simulink model "model_3dof_24"  (R2024b)
settings: Solver=ode4  StartTime=0.0  StopTime=10.0  FixedStep=0.001  RelTol=1e-3
model workspace: external: MATLAB File params.m (data not in the file)
values from neighbouring files (symbols this model uses):
  A = [ ... (first row only)    [params.m]    (also in params_1dof.m; params_3dof.m)
  B = [ ... (first row only)    [params.m]    (also in params_1dof.m = [0; 1/I_xx]; params_3dof.m)
  C = [ ... (first row only)    [params.m]    (also in params_1dof.m = [1 0]; params_3dof.m)
  D = [ ... (first row only)    [params.m]    (also in params_3dof.m)
settings Model: Creator=schwmaxi  LastModifiedBy=schwmaxi
settings OptimizationCC: UseDivisionForNetSlopeComputation=on  GainParamInheritBuiltInType=on  UseFloatMulNetSlope=on  EnhancedBackFolding=on  BooleansAsBitfields=on  PassReuseOutputArgsAs=Individual arguments  StateBitsets=on  DataBitsets=on  ZeroExternalMemoryAtStartup=off  ZeroInternalMemoryAtStartup=off  NoFixptDivByZeroProtection=on  EfficientFloat2IntCast=on  LifeSpan=1  OptimizeBlockOrder=speed  DifferentSizesBufferReuse=on  EfficientTunableParamExpr=on
settings DebuggingCC: ParameterTunabilityLossMsg=error
settings HardwareCC: ProdBitPerPointer=32  ProdBitPerSizeT=32  ProdBitPerPtrDiffT=32  ProdLargestAtomicFloat=None  ProdWordSize=32  ProdLongLongMode=on  ProdHWDeviceType=Custom Processor->Custom Processor
settings SFSimCC: MATLABDynamicMemAlloc=off  SimTargetLang=C++
settings RTWCC: Description=Embedded Coder  SystemTargetFile=ert.tlc  GenCodeOnly=on  TemplateMakefile=ert_default_tmf  TargetLang=C++
settings CodeAppCC: ForceParamTrailComments=on  IgnoreCustomStorageClasses=off  OperatorAnnotations=on  SimulinkDataObjDesc=on  SFDataObjDesc=on  CustomSymbolStrGlobalVar=rt$N$M  CustomSymbolStrType=$N$M  CustomSymbolStrFcn=$N$M$F  CustomSymbolStrMacro=$N$M  InsertBlockDesc=on
settings ERTTargetCC: TargetLangStandard=C++11 (ISO)  GenerateSampleERTMain=on  IncludeMdlTerminateFcn=off  CombineSignalStateStructs=on  SupportAbsoluteTime=off  CodeInterfacePackaging=C++ class  SupportComplex=off  SupportNonInlinedSFcns=on  InlinedParameterPlacement=Hierarchical  RootIOFormat=Structure reference  ERTCustomFileTemplate=example_file_process.tlc  ERTFilePackagingFormat=CompactWithDataFile

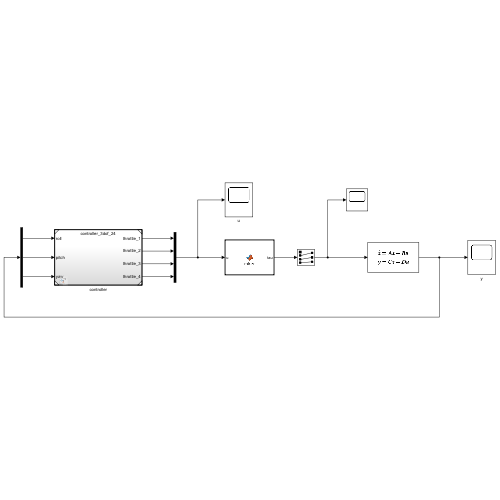
[thumbnail: Simulink's stored preview of the top-level diagram]
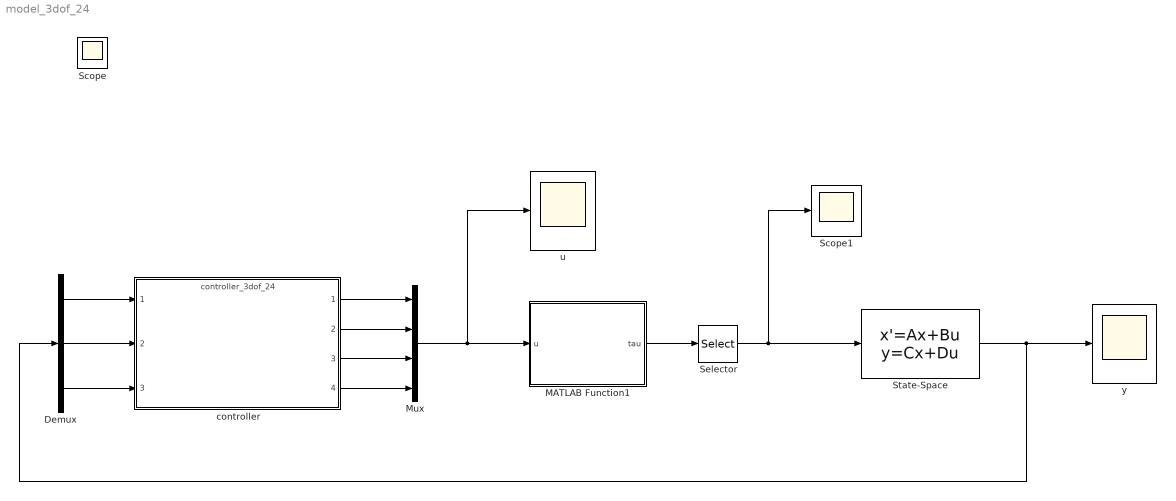
== system model_3dof_24 ==
  Demux : Demux  Outputs=3
  MATLAB Function1 : MATLAB Function  TreatAsAtomicUnit=on
  Mux : Mux
  Scope1 : Scope
  Selector : Selector  InputPortWidth=4  IndexOptions=Index vector (dialog)  Indices=[2 3 4]  OutputSizes=1
  State-Space : StateSpace  A=A  B=B  C=C  D=D  InitialCondition=[0.5, 0, 0, 0, 0, 0]'
  controller : ModelReference  ModelNameDialog=controller_3dof_24.slx  SimulationMode=Normal  ModelReferenceVersion=1.1
  u : Scope
  y : Scope
  Scope : Scope
  wires:
  MATLAB Function1/1(tau) -> Selector/1
  controller/2 -> Mux/2
  controller/1 -> Mux/1
  controller/3 -> Mux/3
  controller/4 -> Mux/4
  Mux/1 -> u/1, MATLAB Function1/1(u)
  Demux/2 -> controller/2
  Demux/1 -> controller/1
  Demux/3 -> controller/3
  Selector/1 -> State-Space/1, Scope1/1
  State-Space/1 -> Demux/1, y/1

== matlab function model_3dof_24/MATLAB Function1 ==
  data: u input; tau output
function tau = mixer(u)
    l = 0.2;
    c = 0.0351;

    E = [
        1 1 1 1;
        0 -l 0 l;
        l 0 -l 0;
        c -c c -c;
    ];

    tau = E * throttle_to_thrust(u);
end

function thrust = throttle_to_thrust(throttle)
    a = 0.0013;
    b = 8.5908;

    thrust = a * (throttle - b).^2;
end
